simulink model "inverted_pendulum_sim"  (R2020b)
settings: Solver=FixedStepAuto  StartTime=0.0  StopTime=20.0  FixedStep=0.001  RelTol=1e-3
values from neighbouring files (symbols this model uses):
  b = 0.1    [inverted_pendulum.m]
  Ftime = 6    [inverted_pendulum.m]
  I = 0.006    [inverted_pendulum.m]
  KD1 = 4    [inverted_pendulum.m]
  KD2 = 1    [inverted_pendulum.m]
  KI1 = 18    [inverted_pendulum.m]
  KP1 = 22    [inverted_pendulum.m]
  KP2 = 2    [inverted_pendulum.m]
  L = 0.3    [inverted_pendulum.m]
  M = 0.5    [inverted_pendulum.m]
  m = 0.2    [inverted_pendulum.m]
  q0 = [0 ; 0]    [inverted_pendulum.m]
  thD = 1*pi    (= 3.14159265359)    [inverted_pendulum.m]
  u0 = [F ; 0]    [inverted_pendulum.m]
  xD = 2    [inverted_pendulum.m]
settings Model: Creator=mymik  LastModifiedBy=mymik

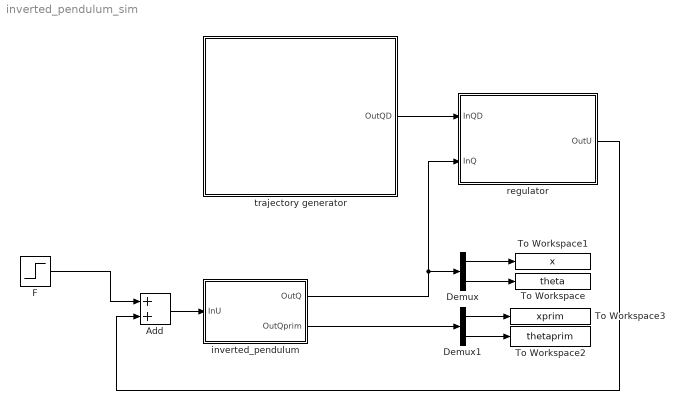
== system inverted_pendulum_sim ==
  Add : Sum
  Demux : Demux  Outputs=2
  Demux1 : Demux  Outputs=2
  F : Step  Time=Ftime  Before=u0  After=[0 ; 0]  SampleTime=0
  To Workspace : ToWorkspace  VariableName=theta  SampleTime=-1
  To Workspace1 : ToWorkspace  VariableName=x  SampleTime=-1
  To Workspace2 : ToWorkspace  VariableName=thetaprim  SampleTime=-1
  To Workspace3 : ToWorkspace  VariableName=xprim  SampleTime=-1
  inverted_pendulum : Subsystem
  regulator : Subsystem
  trajectory generator : Subsystem
  wires:
  trajectory generator/1(OutQD) -> regulator/1(InQD)
  Demux/1 -> To Workspace1/1
  Demux/2 -> To Workspace/1
  inverted_pendulum/1(OutQ) -> Demux/1, regulator/2(InQ)
  inverted_pendulum/2(OutQprim) -> Demux1/1
  Demux1/1 -> To Workspace3/1
  Demux1/2 -> To Workspace2/1
  Add/1 -> inverted_pendulum/1(InU)
  regulator/1(OutU) -> Add/2
  F/1 -> Add/1

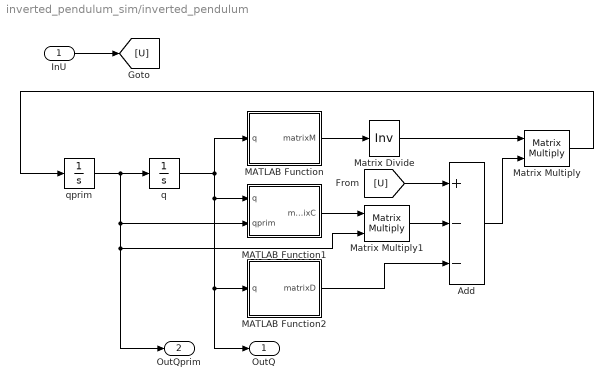
== system inverted_pendulum_sim/inverted_pendulum ==
  InU : Inport
  Add : Sum  Inputs=+--
  MATLAB Function : MATLAB Function  TreatAsAtomicUnit=on
  MATLAB Function1 : MATLAB Function  TreatAsAtomicUnit=on
  MATLAB Function2 : MATLAB Function  TreatAsAtomicUnit=on
  Matrix Divide : Product  Inputs=/  Multiplication=Matrix(*)
  Matrix Multiply : Product  Multiplication=Matrix(*)
  Matrix Multiply1 : Product  Multiplication=Matrix(*)
  q : Integrator  InitialCondition=q0
  qprim : Integrator  InitialCondition=q0
  OutQ : Outport
  OutQprim : Outport  Port=2
  wires:
  MATLAB Function/1(matrixM) -> Matrix Divide/1
  MATLAB Function2/1(matrixD) -> Add/3
  MATLAB Function1/1(matrixC) -> Matrix Multiply1/1
  q/1 -> MATLAB Function1/1(q), OutQ/1, MATLAB Function2/1(q), MATLAB Function/1(q)
  Matrix Multiply/1 -> qprim/1
  Matrix Divide/1 -> Matrix Multiply/1
  [U] -> Add/1
  qprim/1 -> OutQprim/1, Matrix Multiply1/2, MATLAB Function1/2(qprim), q/1
  Matrix Multiply1/1 -> Add/2
  Add/1 -> Matrix Multiply/2
  InU/1 -> [U]

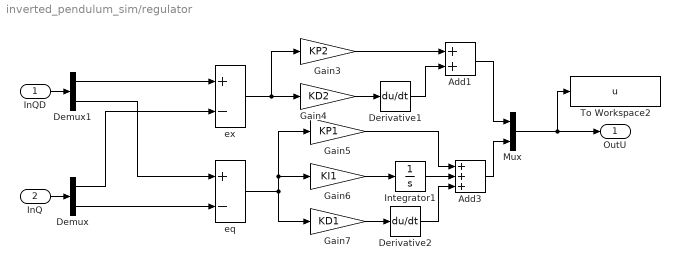
== system inverted_pendulum_sim/regulator ==
  InQD : Inport
  InQ : Inport  Port=2
  Add1 : Sum
  Add3 : Sum  Inputs=+++
  Demux : Demux  Outputs=2
  Demux1 : Demux  Outputs=2
  Derivative1 : Derivative
  Derivative2 : Derivative
  Gain3 : Gain  Gain=KP2
  Gain4 : Gain  Gain=KD2
  Gain5 : Gain  Gain=KP1
  Gain6 : Gain  Gain=KI1
  Gain7 : Gain  Gain=KD1
  Integrator1 : Integrator
  Mux : Mux  Inputs=2
  To Workspace2 : ToWorkspace  VariableName=u  SampleTime=-1
  eq : Sum  Inputs=+-
  ex : Sum  Inputs=+-
  OutU : Outport
  wires:
  InQ/1 -> Demux/1
  Demux/1 -> ex/2
  Demux/2 -> eq/2
  InQD/1 -> Demux1/1
  Demux1/1 -> ex/1
  Demux1/2 -> eq/1
  Gain4/1 -> Derivative1/1
  Derivative1/1 -> Add1/2
  Gain3/1 -> Add1/1
  Mux/1 -> To Workspace2/1, OutU/1
  Gain6/1 -> Integrator1/1
  eq/1 -> Gain5/1, Gain6/1, Gain7/1
  Integrator1/1 -> Add3/2
  Derivative2/1 -> Add3/3
  Gain7/1 -> Derivative2/1
  Gain5/1 -> Add3/1
  ex/1 -> Gain3/1, Gain4/1
  Add3/1 -> Mux/2
  Add1/1 -> Mux/1

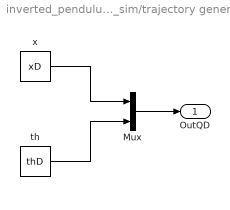
== system inverted_pendulum_sim/trajectory generator ==
  Mux : Mux  Inputs=2
  th : Constant  Value=thD
  x : Constant  Value=xD
  OutQD : Outport
  wires:
  Mux/1 -> OutQD/1
  x/1 -> Mux/1
  th/1 -> Mux/2

== matlab function inverted_pendulum_sim/inverted_pendulum/MATLAB Function1 ==
  data: q input; matrixC output; qprim input; m parameter; b parameter; L parameter
function matrixC = fcn(q, qprim, m, b, L)

C11 = b;
C12 = - m * L * qprim(2) * sin(q(2));
C21 = 0;
C22 = 0;

matrixC = [ C11 , C12 ; C21 , C22 ];

== matlab function inverted_pendulum_sim/inverted_pendulum/MATLAB Function ==
  data: q input; matrixM output; M parameter; m parameter; I parameter; L parameter
function matrixM = fcn(q, M, m, I, L)

M11 = M + m;
M12 = m * L * cos(q(2));
M21 = m * L * cos(q(2));
M22 = I + m * L^2;

matrixM = [ M11 , M12 ; M21 , M22 ];

== matlab function inverted_pendulum_sim/inverted_pendulum/MATLAB Function2 ==
  data: q input; matrixD output; m parameter; L parameter
function matrixD = fcn(q, m, L)

g =  9.80665;

D1 = 0;
D2 = m * g * L * sin(q(2));

matrixD = [ D1 ; D2 ];
